simulink model "mA2_thruster"  (R2023a)
settings: Solver=ode4  StartTime=0.0  StopTime=10.0  FixedStep=0.01  RelTol=1e-3
values from neighbouring files (symbols this model uses):
  AQ = [0.0025,0.0267,0.0016,0.0066,-0.0022,-0.0078,0.0002,0.0061,-0.0016,        -0.0033,0.0012,0.0031,-0.0013,0.0014,0.0009,0.0001,-0.0008,0.0013,0.0012,-0.0001,-0.0007]    [init_mA2_thruster.m]
  AT = [0.0254,0.1782,0.0147,0.0281,-0.0163,-0.0530,0.0006,0.0368,-0.0025,        -0.0177,0.0027,0.0214,-0.0025,0.0012,0.0051,0.0078,-0.0038,0.0035,0.0053,0.0022,-0.0028]    [init_mA2_thruster.m]
  BQ = [0,-0.1108,0.0002,0.0165,-0.0021,0.0085,0.0009,-0.0031,-0.0010,0.0043,        0.0012,0.0001,-0.0008,0.0015,0.0002,-0.0017,0.0005,0.0012,-0.0005,-0.0015,0.0002]    [init_mA2_thruster.m]
  BT = [0,-0.7478,-0.0138,0.1008,-0.0113,0.0472,0.0107,-0.0090,-0.0078,        0.0239,0.0081,-0.0001,-0.0032,0.0093,0.0016,-0.0066,-0.0006,0.0051,-0.0006,-0.0082,-0.0006]    [init_mA2_thruster.m]
  Lx = -2.85    [init_mA2_thruster.m]
  Ly = -0.7    [init_mA2_thruster.m]
  max_angle_displacement = 45    [init_mA2_thruster.m]
  max_rpm = 1200    [init_mA2_thruster.m]
  max_turn_rate = 30    [init_mA2_thruster.m]
  neutral_angle = 45    [init_mA2_thruster.m]
  propeller_diameter = 0.36    [init_mA2_thruster.m]
  servo_time_constant = 0.5    [init_mA2_thruster.m]
libraries: mssSimulink x3, simulink_extras x1
Description:
  | Thruster Fore Stbd
settings Model: Tag=Thruster1  Creator=tobiasvt  LastModifiedBy=HalvorPlatou
settings SolverCC: AlgebraicLoopSolver=TrustRegion
settings DataIOCC: SaveOutput=off  SignalLogging=off  DSMLogging=off  SaveTime=off  ReturnWorkspaceOutputs=off
settings DebuggingCC: UnconnectedInputMsg=warning  UnconnectedOutputMsg=warning  UnconnectedLineMsg=warning
settings ModelReferenceCC: EnableRefExpFcnMdlSchedulingChecks=on
settings SFSimCC: CustomCodeUndefinedFunction=UseInterfaceOnly
settings RTWCC: Description=FMU based on GRT (Functional Mock-up Unit)  SystemTargetFile=grtfmi.tlc  GenerateMakefile=off  TemplateMakefile=none  RetainRTWFile=on
settings STFCustomTargetCC: ConcurrentExecutionCompliant=off  CombineOutputUpdateFcns=on  CodeInterfacePackaging=Reusable function  GRTInterface=off  GenerateAllocFcn=on  UseToolchainInfoCompliant=off  SystemTargetFile=grtfmi.tlc
settings GRTTargetCC: ParMdlRefBuildCompliant=off  CompOptLevelCompliant=off  ConcurrentExecutionCompliant=off  MatFileLogging=off  CodeInterfacePackaging=Reusable function  CPPClassGenCompliant=off  GenerateAllocFcn=on  UseToolchainInfoCompliant=off

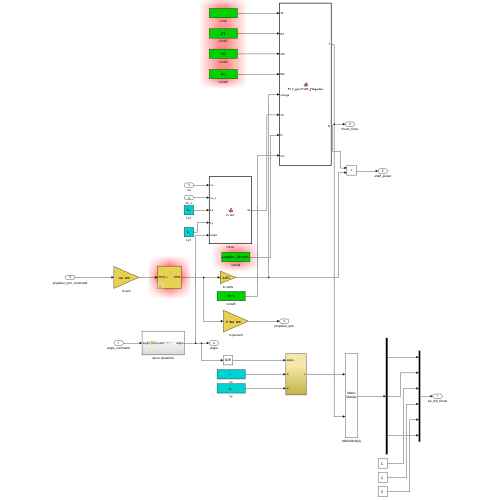
[thumbnail: Simulink's stored preview of the top-level diagram]
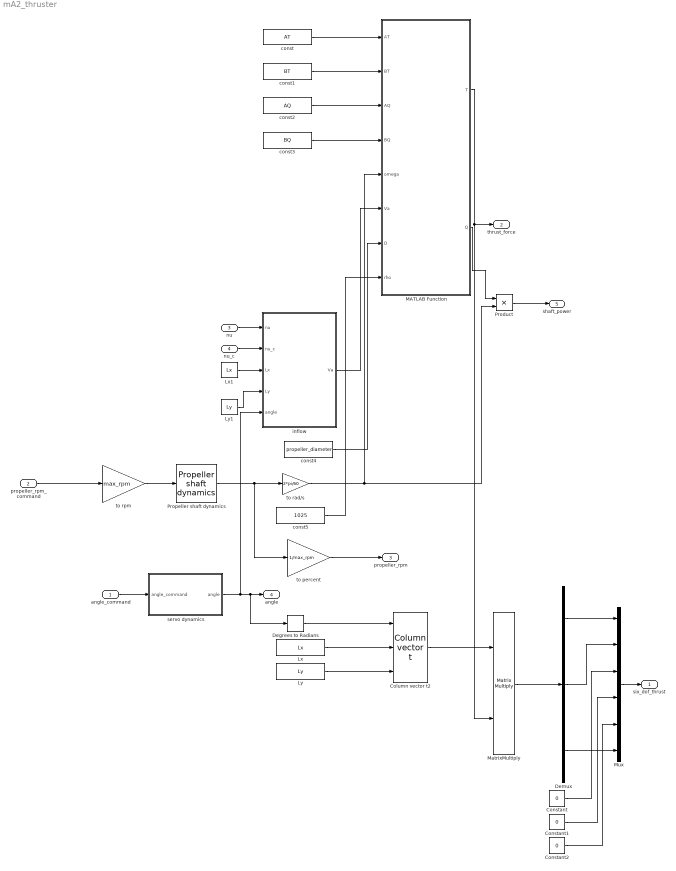
== system mA2_thruster ==
  angle_command : Inport
  propeller_rpm_command : Inport  Port=2
  nu : Inport  Port=3  PortDimensions=6
  nu_c : Inport  Port=4  PortDimensions=6
  Column vector t2 : mssSimulink/Modelling/Propulsion/Actuator Configuration/Column vector t  SystemSampleTime=-1  VariantActivationTime=update diagram  Latency=0  AutoFrameSizeCalculation=off
  Constant : Constant  Value=0
  Constant1 : Constant  Value=0
  Constant2 : Constant  Value=0
  Degrees to Radians : simulink_extras/Transformations/Degrees to Radians
  Demux : Demux  Outputs=3
  Lx : Constant  Value=Lx
  Lx1 : Constant  Value=Lx
  Ly : Constant  Value=Ly
  Ly1 : Constant  Value=Ly
  MATLAB Function : MATLAB Function  TreatAsAtomicUnit=on
  MatrixMultiply : Product  Multiplication=Matrix(*)
  Mux : Mux  Inputs=6
  Product : Product
  Propeller shaft dynamics : mssSimulink/Modelling/Propulsion/Propeller shaft dynamics  rpm_max=max_rpm  rpm_rate=max_rpm_rate  tc=rpm_time_constant
  const : Constant  Value=AT
  const1 : Constant  Value=BT
  const2 : Constant  Value=AQ
  const3 : Constant  Value=BQ
  const4 : Constant  Value=propeller_diameter
  const5 : Constant  Value=1025
  inflow : MATLAB Function  TreatAsAtomicUnit=on
  servo dynamics : Subsystem
  to percent : Gain  Gain=1/max_rpm
  to rad/s : Gain  Gain=2*pi/60
  to rpm : Gain  Gain=max_rpm
  six_dof_thrust : Outport  VectorParamsAs1DForOutWhenUnconnected=off
  thrust_force : Outport  Port=2  VectorParamsAs1DForOutWhenUnconnected=off
  propeller_rpm : Outport  Port=3  VectorParamsAs1DForOutWhenUnconnected=off
  angle : Outport  Port=4  VectorParamsAs1DForOutWhenUnconnected=off
  shaft_power : Outport  Port=5
  wires:
  Ly1/1 -> inflow/4(Ly)
  Lx1/1 -> inflow/3(Lx)
  to percent/1 -> propeller_rpm/1
  angle_command/1 -> servo dynamics/1(angle_command)
  Demux/3 -> Mux/6
  Constant1/1 -> Mux/4
  Constant/1 -> Mux/3
  Propeller shaft dynamics/1 -> to percent/1, to rad/s/1
  Degrees to Radians/1 -> Column vector t2/1
  to rpm/1 -> Propeller shaft dynamics/1
  propeller_rpm_command/1 -> to rpm/1
  MatrixMultiply/1 -> Demux/1
  Demux/2 -> Mux/2
  inflow/1(Va) -> MATLAB Function/6(Va)
  Ly/1 -> Column vector t2/3
  Column vector t2/1 -> MatrixMultiply/1
  Constant2/1 -> Mux/5
  Lx/1 -> Column vector t2/2
  nu_c/1 -> inflow/2(nu_c)
  Mux/1 -> six_dof_thrust/1
  nu/1 -> inflow/1(nu)
  const1/1 -> MATLAB Function/2(BT)
  const3/1 -> MATLAB Function/4(BQ)
  const/1 -> MATLAB Function/1(AT)
  const2/1 -> MATLAB Function/3(AQ)
  MATLAB Function/2(Q) -> Product/1
  const5/1 -> MATLAB Function/8(rho)
  const4/1 -> MATLAB Function/7(D)
  Demux/1 -> Mux/1
  Product/1 -> shaft_power/1
  to rad/s/1 -> MATLAB Function/5(omega), Product/2
  MATLAB Function/1(T) -> MatrixMultiply/2, thrust_force/1
  servo dynamics/1(angle) -> angle/1, Degrees to Radians/1, inflow/5(angle)

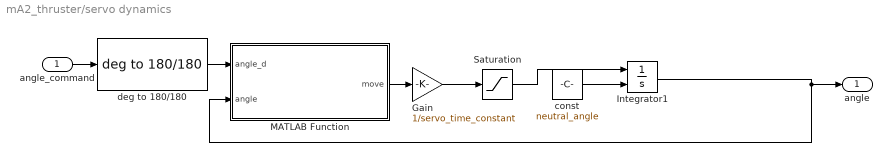
== system mA2_thruster/servo dynamics ==
  angle_command : Inport
  Gain : Gain  Gain=1/servo_time_constant  SaturateOnIntegerOverflow=on  OutDataTypeStr=Inherit: Same as input  ParamDataTypeStr=Inherit: Same as input
  Integrator1 : Integrator  InitialConditionSource=external  InitialCondition=neutral_angle  LimitOutput=on  UpperSaturationLimit=neutral_angle + max_angle_displacement  LowerSaturationLimit=neutral_angle - max_angle_displacement
  MATLAB Function : MATLAB Function  TreatAsAtomicUnit=on
  Saturation : Saturate  UpperLimit=max_turn_rate  LowerLimit=-max_turn_rate
  const : Constant  Value=neutral_angle
  deg to 180/180 : mssSimulink/Utilities/Math Operations/deg to 180//180
  angle : Outport
  wires:
  Saturation/1 -> Integrator1/1
  MATLAB Function/1(move) -> Gain/1
  Gain/1 -> Saturation/1
  angle_command/1 -> deg to 180/180/1
  Integrator1/1 -> MATLAB Function/2(angle), angle/1
  deg to 180/180/1 -> MATLAB Function/1(angle_d)
  const/1 -> Integrator1/2

== matlab function mA2_thruster/MATLAB Function ==
  data: AT input; T output; BT input; AQ input; BQ input; omega input; Va input; D input; rho input; Q output
function [T, Q] = four_quadrant_propeller(AT,BT,AQ,BQ,omega,Va,D,rho)
    beta = atan2(Va,0.7*omega*D*0.5);
    CT = 0; CQ = 0;
    for k = 0:length(AT)-1
        CT = CT + AT(k+1)*cos(beta*k) + BT(k+1)*sin(beta*k);
        CQ = CQ + AQ(k+1)*cos(beta*k) + BQ(k+1)*sin(beta*k);
    end
    T = (pi*D^2*rho*CT/8.0)*(Va^2 + (0.7*omega*0.5*D)^2);
    Q = (pi*D^3*rho*CQ/8.0)*(Va^2 + (0.7*omega*0.5*D)^2);
end

== matlab function mA2_thruster/inflow ==
  data: nu input; Va output; nu_c input; Lx input; Ly input; angle input
function Va = inflow(nu, nu_c, Lx, Ly, angle)
    v_T = [nu(1) - Ly*nu(6); nu(2) + Lx*nu(6)];%Velocity of thruster
    v_Tr = v_T - nu_c(1:2);%Velocity of thruster through water
    Va = v_Tr(1)*cos(deg2rad(angle)) + v_Tr(2)*sin(deg2rad(angle)); 
end

== matlab function mA2_thruster/servo dynamics/MATLAB Function ==
  data: angle_d input; move output; angle input
function move = shortest_angle_path(angle_d, angle)
    diff = mod(angle_d - angle + 180, 360) - 180;
    if diff < -180
        move = diff + 360;
    else
        move = diff;
    end
end
